simulink model "Saturation_Limit"  (Simulink 8.0)
settings: Solver=ode45  StartTime=0.0  StopTime=10.0  RelTol=1e-3
libraries: simulink x1
settings Model: Creator=Faradars  LastModifiedBy=Faradars

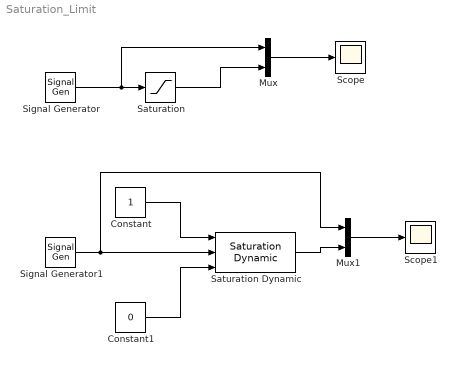
== system Saturation_Limit ==
  Constant : Constant
  Constant1 : Constant  Value=0
  Mux : Mux  Inputs=2
  Mux1 : Mux  Inputs=2
  Saturation : Saturate
  Saturation Dynamic : simulink/Discontinuities/Saturation Dynamic  OutMin=[]  OutMax=[]  OutDataTypeStr=Inherit: Same as second input  OutDataType=fixdt(1, 16)  OutScaling=2^-10  DoSatur=off
  Scope : Scope
  Scope1 : Scope
  Signal Generator : SignalGenerator  Frequency=0.25
  Signal Generator1 : SignalGenerator  Frequency=0.25
  wires:
  Mux/1 -> Scope/1
  Saturation/1 -> Mux/2
  Signal Generator/1 -> Mux/1, Saturation/1
  Constant/1 -> Saturation Dynamic/1
  Constant1/1 -> Saturation Dynamic/3
  Signal Generator1/1 -> Saturation Dynamic/2, Mux1/1
  Mux1/1 -> Scope1/1
  Saturation Dynamic/1 -> Mux1/2
